simulink model "ComparingControllers"  (R2017b)
settings: Solver=VariableStepAuto  StartTime=0.0  StopTime=1000  RelTol=1e-3
libraries: simulink x2
settings Model: Creator=shayan  LastModifiedBy=shayan

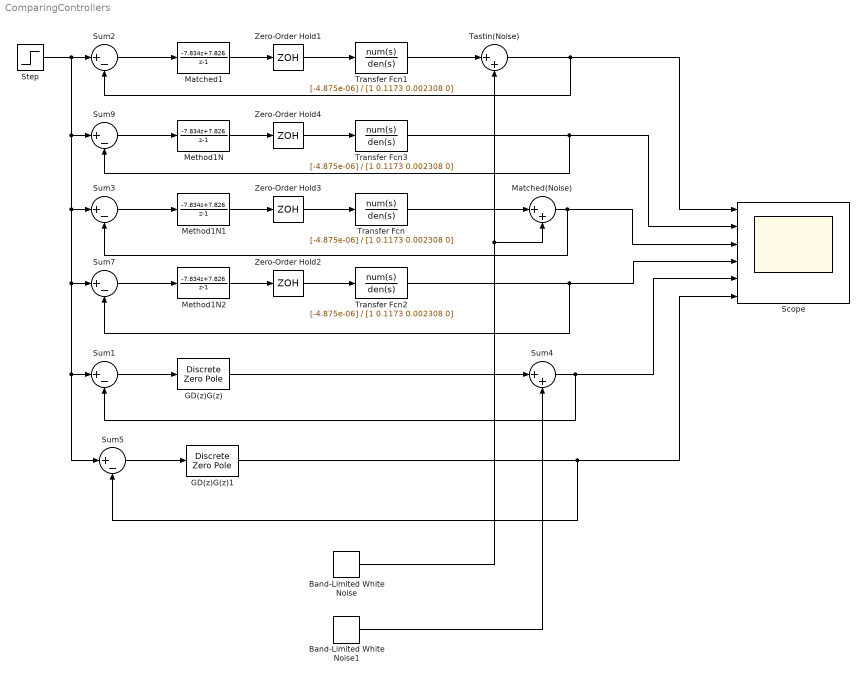
== system ComparingControllers ==
  Band-Limited White Noise : simulink/Sources/Band-Limited White Noise  Cov=[0.01]  Ts=4  seed=[23341]
  Band-Limited White Noise1 : simulink/Sources/Band-Limited White Noise  Cov=[0.01]  Ts=10  seed=[23341]
  GD(z)G(z) : DiscreteZeroPole  Zeros=[-2.8306 -0.1967]  Poles=[0.7788 0.4920 0.3972]  Gain=0.0197  SampleTime=10
  GD(z)G(z)1 : DiscreteZeroPole  Zeros=[-2.8306 -0.1967]  Poles=[0.7788 0.4920 0.3972]  Gain=0.0197  SampleTime=10
  Matched(Noise) : Sum  Inputs=|++
  Matched1 : DiscreteTransferFcn  Numerator=[-7.834 7.826]  Denominator=[1 -1]  SampleTime=4
  Method1N : DiscreteTransferFcn  Numerator=[-7.834 7.826]  Denominator=[1 -1]  SampleTime=4
  Method1N1 : DiscreteTransferFcn  Numerator=[-7.834 7.826]  Denominator=[1 -1]  SampleTime=4
  Method1N2 : DiscreteTransferFcn  Numerator=[-7.834 7.826]  Denominator=[1 -1]  SampleTime=4
  Scope : Scope  NumInputPorts=6
  Step : Step  SampleTime=0
  Sum{1..3,5,7,9} (6 alike) : Sum  Inputs=|+-
  Sum4 : Sum  Inputs=|++
  Tastin(Noise) : Sum  Inputs=|++
  Transfer Fcn{,1..3} (4 alike) : TransferFcn  Numerator=[-4.875e-06]  Denominator=[1 0.1173 0.002308 0]
  Zero-Order Hold{1..4} (4 alike) : ZeroOrderHold  SampleTime=4
  wires:
  Sum1/1 -> GD(z)G(z)/1
  Step/1 -> Sum7/1, Sum5/1, Sum1/1, Sum3/1, Sum9/1, Sum2/1
  Sum3/1 -> Method1N1/1
  Method1N1/1 -> Zero-Order Hold3/1
  Zero-Order Hold3/1 -> Transfer Fcn/1
  Matched1/1 -> Zero-Order Hold1/1
  Zero-Order Hold1/1 -> Transfer Fcn1/1
  Sum2/1 -> Matched1/1
  Transfer Fcn/1 -> Matched(Noise)/1
  GD(z)G(z)/1 -> Sum4/1
  Sum4/1 -> Scope/5, Sum1/2
  Sum5/1 -> GD(z)G(z)1/1
  GD(z)G(z)1/1 -> Sum5/2, Scope/6
  Sum7/1 -> Method1N2/1
  Method1N2/1 -> Zero-Order Hold2/1
  Zero-Order Hold2/1 -> Transfer Fcn2/1
  Zero-Order Hold4/1 -> Transfer Fcn3/1
  Method1N/1 -> Zero-Order Hold4/1
  Sum9/1 -> Method1N/1
  Transfer Fcn1/1 -> Tastin(Noise)/1
  Band-Limited White Noise/1 -> Matched(Noise)/2, Tastin(Noise)/2
  Transfer Fcn2/1 -> Sum7/2, Scope/4
  Matched(Noise)/1 -> Sum3/2, Scope/3
  Transfer Fcn3/1 -> Scope/2, Sum9/2
  Tastin(Noise)/1 -> Scope/1, Sum2/2
  Band-Limited White Noise1/1 -> Sum4/2
